simulink subsystem "SimulinkPlantModels"  (R2023b)
settings: Solver=VariableStepAuto  StartTime=0.0  StopTime=10.0  RelTol=1e-3
undefined symbols (not defined in the file): PlntTrnsfrCaseAxlSpdLock, PlntTrnsfrCaseTrqSplitRatio
libraries: simulink x2
settings Model: ModifiedByFormat=The MathWorks, Inc.  Creator=The MathWorks, Inc.  LastModifiedBy=The MathWorks, Inc.
settings DebuggingCC: SubsystemReferenceDiagnosticForUnitTest=warning

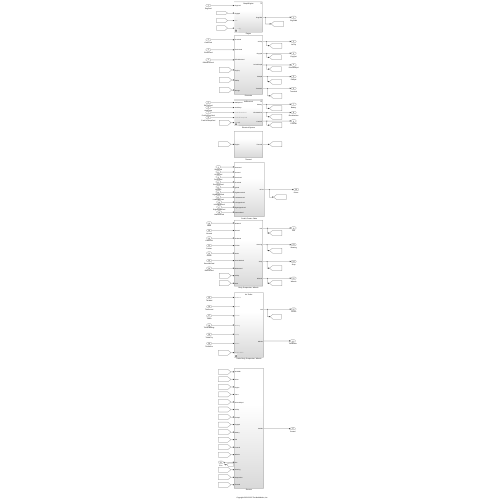
[thumbnail: Simulink's stored preview of the top-level diagram]
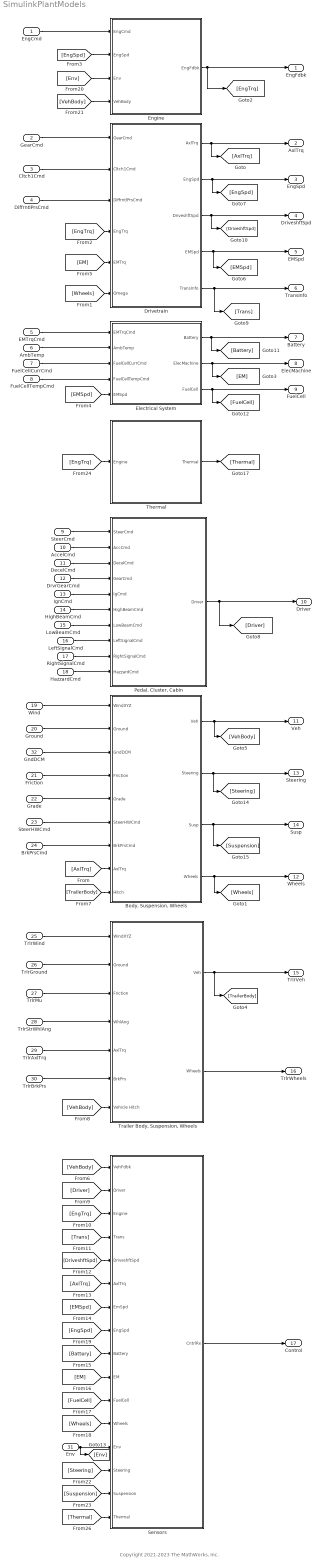
== system SimulinkPlantModels ==
  note: Copyright 2021-2023 The MathWorks, Inc.
  EngCmd : Inport
  GearCmd : Inport  Port=2
  Cltch1Cmd : Inport  Port=3
  DiffrntlPrsCmd : Inport  Port=4
  EMTrqCmd : Inport  Port=5
  AmbTemp : Inport  Port=6
  FuelCellCurrCmd : Inport  Port=7
  FuelCellTempCmd : Inport  Port=8
  SteerCmd : Inport  Port=9
  AccelCmd : Inport  Port=10
  DecelCmd : Inport  Port=11
  DrvrGearCmd : Inport  Port=12
  IgnCmd : Inport  Port=13
  HighBeamCmd : Inport  Port=14
  LowBeamCmd : Inport  Port=15
  LeftSignalCmd : Inport  Port=16
  RightSignalCmd : Inport  Port=17
  HazzardCmd : Inport  Port=18
  Wind : Inport  Port=19
  Ground : Inport  Port=20
  Friction : Inport  Port=21
  Grade : Inport  Port=22
  SteerHWCmd : Inport  Port=23
  BrkPrsCmd : Inport  Port=24
  TrlrWind : Inport  Port=25
  TrlrGround : Inport  Port=26
  TrlrMu : Inport  Port=27
  TrlrStrWhlAng : Inport  Port=28
  TrlrAxlTrq : Inport  Port=29
  TrlrBrkPrs : Inport  Port=30
  Env : Inport  Port=31
  GndDCM : Inport  Port=32
  "Body, Suspension, Wheels" : Subsystem  VariantControl=Lateral Vehicle Dynamics
  Drivetrain : Subsystem
  Electrical System : Subsystem  Variant=on  VariantChoicesSpecifier={'ElectricalSystem', 'NoElectrical'}  VariantControlMode=label  VariantControl=Choice  LabelModeActiveChoice=NoElectrical
  Engine : Subsystem  Variant=on  VariantChoicesSpecifier={'CiEngine', 'CiMappedEngine', 'FMUEngine', 'NoEngine', 'SiDLEngine', 'SiEngine', 'SiMappedEngine', 'SimpleEngine'}  VariantControlMode=label  LabelModeActiveChoice=SimpleEngine
  "Pedal, Cluster, Cabin" : Subsystem
  Sensors : Subsystem
  Thermal : Subsystem
  "Trailer Body, Suspension, Wheels" : Subsystem  Variant=on  VariantControlMode=label  LabelModeActiveChoice=No Trailer
  EngFdbk : Outport
  AxlTrq : Outport  Port=2
  EngSpd : Outport  Port=3
  DriveshftSpd : Outport  Port=4
  EMSpd : Outport  Port=5
  TransInfo : Outport  Port=6
  Battery : Outport  Port=7
  ElecMachine : Outport  Port=8
  FuelCell : Outport  Port=9
  Driver : Outport  Port=10
  Veh : Outport  Port=11
  Wheels : Outport  Port=12
  Steering : Outport  Port=13
  Susp : Outport  Port=14
  TrlrVeh : Outport  Port=15
  TrlrWheels : Outport  Port=16
  Control : Outport  Port=17
  wires:
  "Body, Suspension, Wheels"/2(Steering) -> [Steering], Steering/1
  [Suspension] -> Sensors/15(Suspension)
  "Body, Suspension, Wheels"/3(Susp) -> [Suspension], Susp/1
  [Steering] -> Sensors/14(Steering)
  Drivetrain/5(TransInfo) -> TransInfo/1, [Trans]
  Sensors/1(CntrlRx) -> Control/1
  Grade/1 -> "Body, Suspension, Wheels"/5(Grade)
  [EngTrq] -> Sensors/3(Engine)
  IgnCmd/1 -> "Pedal, Cluster, Cabin"/5(IgCmd)
  GndDCM/1 -> "Body, Suspension, Wheels"/3(GndDCM)
  Env/1 -> Sensors/13(Env), [Env]
  [EMSpd] -> Electrical System/5(EMSpd)
  EngCmd/1 -> Engine/1(EngCmd)
  Engine/1(EngFdbk) -> EngFdbk/1, [EngTrq]
  DiffrntlPrsCmd/1 -> Drivetrain/3(DiffrntlPrsCmd)
  [Env] -> Engine/3(Env)
  [VehBody] -> Engine/4(VehBody)
  [Battery] -> Sensors/9(Battery)
  [EngSpd] -> Sensors/8(EngSpd)
  [EngSpd] -> Engine/2(EngSpd)
  [Trans] -> Sensors/4(Trans)
  [Wheels] -> Sensors/12(Wheels)
  [EMSpd] -> Sensors/7(EmSpd)
  [EM] -> Sensors/10(EM)
  BrkPrsCmd/1 -> "Body, Suspension, Wheels"/7(BrkPrsCmd)
  FuelCellCurrCmd/1 -> Electrical System/3(FuelCellCurrCmd)
  [DriveshftSpd] -> Sensors/5(DriveshftSpd)
  [FuelCell] -> Sensors/11(FuelCell)
  [Driver] -> Sensors/2(Driver)
  "Trailer Body, Suspension, Wheels"/1(Veh) -> TrlrVeh/1, [TrailerBody]
  "Trailer Body, Suspension, Wheels"/2(Wheels) -> TrlrWheels/1
  Electrical System/2(ElecMachine) -> ElecMachine/1, [EM]
  [TrailerBody] -> "Body, Suspension, Wheels"/9(Hitch)
  "Body, Suspension, Wheels"/4(Wheels) -> [Wheels], Wheels/1
  "Pedal, Cluster, Cabin"/1(Driver) -> Driver/1, [Driver]
  Ground/1 -> "Body, Suspension, Wheels"/2(Ground)
  [VehBody] -> Sensors/1(VehFdbk)
  [Wheels] -> Drivetrain/6(Omega)
  GearCmd/1 -> Drivetrain/1(GearCmd)
  [EM] -> Drivetrain/5(EMTrq)
  Drivetrain/4(EMSpd) -> EMSpd/1, [EMSpd]
  [EngTrq] -> Drivetrain/4(EngTrq)
  AccelCmd/1 -> "Pedal, Cluster, Cabin"/2(AccCmd)
  EMTrqCmd/1 -> Electrical System/1(EMTrqCmd)
  Drivetrain/1(AxlTrq) -> AxlTrq/1, [AxlTrq]
  TrlrAxlTrq/1 -> "Trailer Body, Suspension, Wheels"/5(AxlTrq)
  Wind/1 -> "Body, Suspension, Wheels"/1(WindXYZ)
  TrlrStrWhlAng/1 -> "Trailer Body, Suspension, Wheels"/4(WhlAng)
  Friction/1 -> "Body, Suspension, Wheels"/4(Friction)
  FuelCellTempCmd/1 -> Electrical System/4(FuelCellTempCmd)
  [AxlTrq] -> "Body, Suspension, Wheels"/8(AxlTrq)
  TrlrWind/1 -> "Trailer Body, Suspension, Wheels"/1(WindXYZ)
  Drivetrain/3(DriveshftSpd) -> DriveshftSpd/1, [DriveshftSpd]
  SteerCmd/1 -> "Pedal, Cluster, Cabin"/1(SteerCmd)
  AmbTemp/1 -> Electrical System/2(AmbTemp)
  Cltch1Cmd/1 -> Drivetrain/2(Cltch1Cmd)
  DecelCmd/1 -> "Pedal, Cluster, Cabin"/3(DecelCmd)
  TrlrMu/1 -> "Trailer Body, Suspension, Wheels"/3(Friction)
  Drivetrain/2(EngSpd) -> EngSpd/1, [EngSpd]
  DrvrGearCmd/1 -> "Pedal, Cluster, Cabin"/4(GearCmd)
  [AxlTrq] -> Sensors/6(AxlTrq)
  SteerHWCmd/1 -> "Body, Suspension, Wheels"/6(SteerHWCmd)
  TrlrBrkPrs/1 -> "Trailer Body, Suspension, Wheels"/6(BrkPrs)
  [VehBody] -> "Trailer Body, Suspension, Wheels"/7(Vehicle Hitch)
  "Body, Suspension, Wheels"/1(Veh) -> Veh/1, [VehBody]
  Electrical System/3(FuelCell) -> FuelCell/1, [FuelCell]
  TrlrGround/1 -> "Trailer Body, Suspension, Wheels"/2(Ground)
  Electrical System/1(Battery) -> Battery/1, [Battery]
  Thermal/1(Thermal) -> [Thermal]
  [EngTrq] -> Thermal/1(Engine)
  [Thermal] -> Sensors/16(Thermal)
  RightSignalCmd/1 -> "Pedal, Cluster, Cabin"/9(RightSignalCmd)
  LowBeamCmd/1 -> "Pedal, Cluster, Cabin"/7(LowBeamCmd)
  HighBeamCmd/1 -> "Pedal, Cluster, Cabin"/6(HighBeamCmd)
  HazzardCmd/1 -> "Pedal, Cluster, Cabin"/10(HazzardCmd)
  LeftSignalCmd/1 -> "Pedal, Cluster, Cabin"/8(LeftSignalCmd)

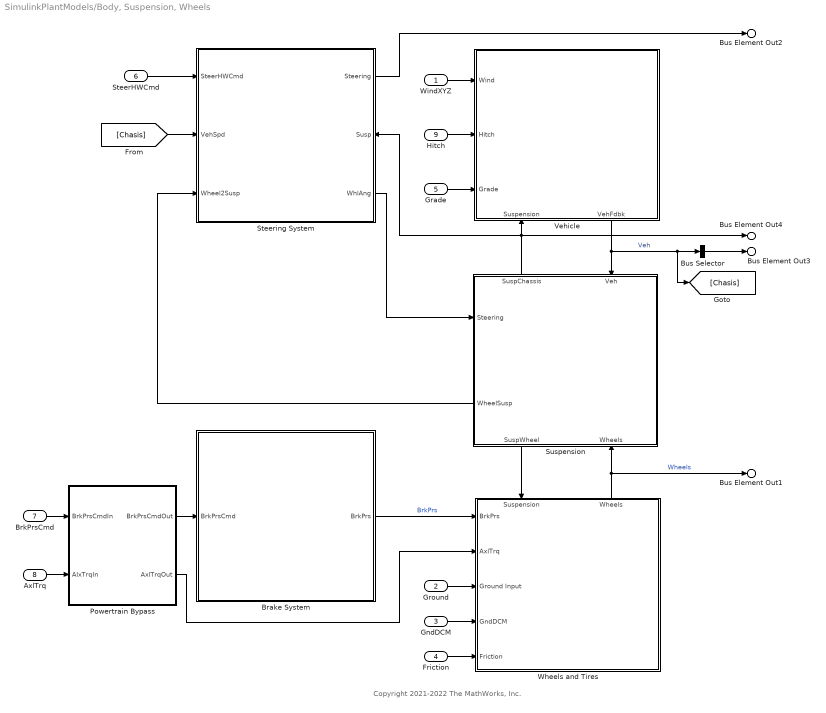
== system SimulinkPlantModels/Body, Suspension, Wheels ==
  note: Copyright 2021-2022 The MathWorks, Inc.
  WindXYZ : Inport  Unit=m/s  PortDimensions=3
  Ground : Inport  Port=2  Unit=m  PortDimensions=4
  GndDCM : Inport  Port=3
  Friction : Inport  Port=4  Unit=1  PortDimensions=4
  Grade : Inport  Port=5
  SteerHWCmd : Inport  Port=6  Unit=rad
  BrkPrsCmd : Inport  Port=7  PortDimensions=4
  AxlTrq : Inport  Port=8  Unit=N*m  PortDimensions=4
  Hitch : Inport  Port=9
  Brake System : Subsystem  Variant=on  VariantControlMode=label  VariantControl=Choice  LabelModeActiveChoice=BrakingHydraulics
      mask Display: disp('Brake System');
  Bus Selector : BusSelector  OutputSignals=InertFrm,BdyFrm  OutputAsBus=on
  Powertrain Bypass : Subsystem  Variant=on  VariantControlMode=label  VariantControl=Choice  LabelModeActiveChoice=Pass Through
  Steering System : Subsystem  Variant=on  VariantChoicesSpecifier={'DynamicSteering', 'KinematicSteering', 'MappedSteering', 'NoSteering', 'SteeringSystem'}  VariantControlMode=label  VariantControl=0  LabelModeActiveChoice=NoSteering
      settings: PortSchema="{\"entries\":[{\"content\":{\"sides\":[{\"content\":{\"connectorIds\":[\"In1\",\"In2\",\"In3\"]},\"type\":\"ConnectorPlacement.EquallySpacedRectSide\",\"uuid\":\"f4eae9a1-ee72-4894-9c3f-d81ee40fba89\"},{\"content\":{\"connectorIds\":[\"Out1\",\"In4\",\"Out2\"],\"side\":\"RIGHT\"},\"type\":\"ConnectorPlacement.EquallySpacedRectSide\",\"uuid\":\"c62a78d9-dc5d-4f96-a554-c82d7fa22a9e\"},{\"content\":{\"connectorIds\":[],\"side\":\"TOP\"},\"type\":\"ConnectorPlacement.EquallySpacedRectSide\",\"uuid\":\"38f3851a-1d1e-4a2b-8c09-8e5c8dcc7723\"}]},\"type\":\"ConnectorPlacement.EquallySpacedConnector\",\"uuid\":\"9f269846-92fa-4948-bc2b-71154f41fdde\"}],\"packageUris\":[\"http://schema.mathworks.com/mf0/Connector/R2020b\"],\"version\":\"1.0\"}"
      mask Display: disp('Steering System');
  Suspension : Subsystem  Variant=on  VariantChoicesSpecifier={'KinematicsComplianceIndependentSuspension', 'KinematicsComplianceTwistBeamSuspension', 'MacPhersonFrontSuspensionSolidAxleRearSuspension', 'NoSuspension'}  VariantControlMode=label  VariantControl=Choice  LabelModeActiveChoice=NoSuspension
      settings: PortSchema="{\"entries\":[{\"content\":{\"sides\":[{\"content\":{\"connectorIds\":[\"In1\",\"Out3\"]},\"type\":\"ConnectorPlacement.EquallySpacedRectSide\",\"uuid\":\"0a9265e3-f55e-4b74-9b74-681dc9522591\"},{\"content\":{\"connectorIds\":[],\"side\":\"RIGHT\"},\"type\":\"ConnectorPlacement.EquallySpacedRectSide\",\"uuid\":\"92df639a-7bc2-4e90-97ea-0cb216e2f16a\"},{\"content\":{\"connectorIds\":[\"Out2\",\"In2\"],\"side\":\"TOP\"},\"type\":\"ConnectorPlacement.EquallySpacedRectSide\",\"uuid\":\"2064b6cb-c7a8-4cfb-82de-a07750d990cb\"},{\"content\":{\"connectorIds\":[\"Out1\",\"In3\"],\"side\":\"BOTTOM\"},\"type\":\"ConnectorPlacement.EquallySpacedRectSide\",\"uuid\":\"169bd4e6-c3fe-4e36-acea-c25875014463\"}]},\"type\":\"ConnectorPlacement.EquallySpacedConnector\",\"uuid\":\"e0b50182-0637-4594-80e7-4ddd0df85797\"}],\"packageUris\":[\"http://schema.mathworks.com/mf0/Connector/R2020b\"],\"version\":\"1.0\"}"
      mask Display: disp('Suspension');
  Vehicle : Subsystem  Variant=on  VariantChoicesSpecifier={'VehicleBody1DOFLongitudinal', 'VehicleBody3DOFLongitudinal', 'VehicleBody6DOF'}  VariantControlMode=label  VariantControl=Choice  LabelModeActiveChoice=VehicleBody3DOFLongitudinal
      settings: PortSchema="{\"entries\":[{\"content\":{\"sides\":[{\"content\":{\"connectorIds\":[\"In1\",\"In2\",\"In3\"]},\"type\":\"ConnectorPlacement.EquallySpacedRectSide\",\"uuid\":\"0a9265e3-f55e-4b74-9b74-681dc9522591\"},{\"content\":{\"connectorIds\":[],\"side\":\"RIGHT\"},\"type\":\"ConnectorPlacement.EquallySpacedRectSide\",\"uuid\":\"92df639a-7bc2-4e90-97ea-0cb216e2f16a\"},{\"content\":{\"connectorIds\":[],\"side\":\"TOP\"},\"type\":\"ConnectorPlacement.EquallySpacedRectSide\",\"uuid\":\"2064b6cb-c7a8-4cfb-82de-a07750d990cb\"},{\"content\":{\"connectorIds\":[\"In4\",\"Out1\"],\"side\":\"BOTTOM\"},\"type\":\"ConnectorPlacement.EquallySpacedRectSide\",\"uuid\":\"2b34afca-0a88-43db-924f-6476183b84bd\"}]},\"type\":\"ConnectorPlacement.EquallySpacedConnector\",\"uuid\":\"e0b50182-0637-4594-80e7-4ddd0df85797\"}],\"packageUris\":[\"http://schema.mathworks.com/mf0/Connector/R2020b\"],\"version\":\"1.0\"}"
      mask Display: disp('Vehicle Body');
  Wheels and Tires : Subsystem  Variant=on  VariantChoicesSpecifier={'CombinedSlipTiresLongitudinal', 'DugoffTires', 'FialaTires', 'MFTires', 'MFTiresLongitudinal'}  VariantControlMode=label  VariantControl=Choice  LabelModeActiveChoice=MFTiresLongitudinal
      settings: PortSchema="{\"entries\":[{\"content\":{\"sides\":[{\"content\":{\"connectorIds\":[\"In1\",\"In2\",\"In3\",\"In4\",\"In5\"]},\"type\":\"ConnectorPlacement.EquallySpacedRectSide\",\"uuid\":\"fdb4d4cd-d0c0-42d9-b073-775af31e96a1\"},{\"content\":{\"connectorIds\":[],\"side\":\"RIGHT\"},\"type\":\"ConnectorPlacement.EquallySpacedRectSide\",\"uuid\":\"04106ddf-9917-4cd4-b177-ae763d642686\"},{\"content\":{\"connectorIds\":[\"In6\",\"Out1\"],\"side\":\"TOP\"},\"type\":\"ConnectorPlacement.EquallySpacedRectSide\",\"uuid\":\"568bf95c-0e25-4c45-a134-c198357b75be\"}]},\"type\":\"ConnectorPlacement.EquallySpacedConnector\",\"uuid\":\"4f44df5e-0d14-43ea-934e-2abe86546e95\"}],\"packageUris\":[\"http://schema.mathworks.com/mf0/Connector/R2020b\"],\"version\":\"1.0\"}"
      mask Display: disp('Wheels and Tires');
  Bus Element Out3 : Outport  PortName=Veh
  Bus Element Out2 : Outport  Port=2  PortName=Steering
  Bus Element Out4 : Outport  Port=3  PortName=Susp
  Bus Element Out1 : Outport  Port=4  PortName=Wheels
  wires:
  GndDCM/1 -> Wheels and Tires/4(GndDCM)
  Friction/1 -> Wheels and Tires/5(Friction)
  Powertrain Bypass/2(AxlTrqOut) -> Wheels and Tires/2(AxlTrq)
  Ground/1 -> Wheels and Tires/3(Ground Input)
  Grade/1 -> Vehicle/3(Grade)
  Wheels and Tires/1(Wheels) -> Bus Element Out1/1, Suspension/3(Wheels)  "Wheels"
  Suspension/1(SuspWheel) -> Wheels and Tires/6(Suspension)
  Brake System/1(BrkPrs) -> Wheels and Tires/1(BrkPrs)  "BrkPrs"
  Vehicle/1(VehFdbk) -> [Chasis], Bus Selector/1, Suspension/2(Veh)  "Veh"
  Hitch/1 -> Vehicle/2(Hitch)
  WindXYZ/1 -> Vehicle/1(Wind)
  Suspension/2(SuspChassis) -> Steering System/4(Susp), Bus Element Out4/1, Vehicle/4(Suspension)
  Steering System/2(WhlAng) -> Suspension/1(Steering)
  BrkPrsCmd/1 -> Powertrain Bypass/1(BrkPrsCmdIn)
  Bus Selector/1 -> Bus Element Out3/1
  [Chasis] -> Steering System/2(VehSpd)
  SteerHWCmd/1 -> Steering System/1(SteerHWCmd)
  Steering System/1(Steering) -> Bus Element Out2/1
  Powertrain Bypass/1(BrkPrsCmdOut) -> Brake System/1(BrkPrsCmd)
  AxlTrq/1 -> Powertrain Bypass/2(AlxTrqIn)
  Suspension/3(WheelSusp) -> Steering System/3(Wheel2Susp)

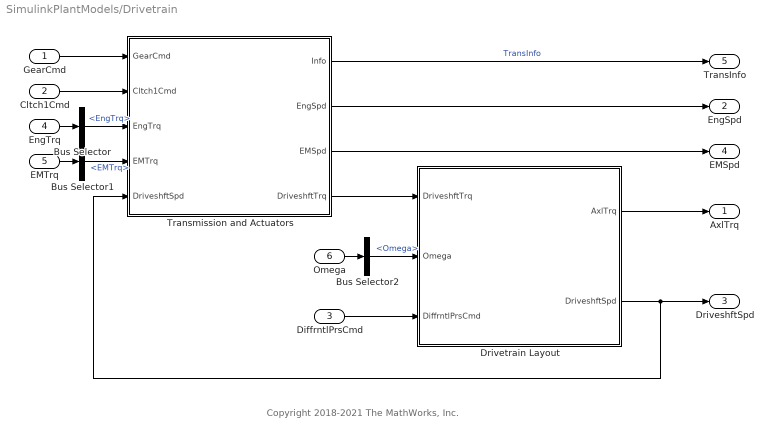
== system SimulinkPlantModels/Drivetrain ==
  note: Copyright 2018-2021 The MathWorks, Inc.
  GearCmd : Inport
  Cltch1Cmd : Inport  Port=2
  DiffrntlPrsCmd : Inport  Port=3
  EngTrq : Inport  Port=4
  EMTrq : Inport  Port=5
  Omega : Inport  Port=6
  Bus Selector : BusSelector  OutputSignals=EngTrq
  Bus Selector1 : BusSelector  OutputSignals=EMTrq
  Bus Selector2 : BusSelector  OutputSignals=Wheels.Omega
  Drivetrain Layout : Subsystem  VariantControl=New
  Transmission and Actuators : Subsystem  Variant=on  VariantChoicesSpecifier={'BEV1EM', 'BEV2EM', 'BEV3EM', 'BEV4EM', 'ConventionalVehicle', 'HEVIPS', 'HEVMM', 'HEVP0', 'HEVP1', 'HEVP2', 'HEVP3', 'HEVP4'}  VariantControlMode=label  LabelModeActiveChoice=ConventionalVehicle
  AxlTrq : Outport  VectorParamsAs1DForOutWhenUnconnected=off
  EngSpd : Outport  Port=2  Unit=rad/s  VectorParamsAs1DForOutWhenUnconnected=off
  DriveshftSpd : Outport  Port=3  VectorParamsAs1DForOutWhenUnconnected=off
  EMSpd : Outport  Port=4  Unit=rad/s  VectorParamsAs1DForOutWhenUnconnected=off
  TransInfo : Outport  Port=5  VectorParamsAs1DForOutWhenUnconnected=off
  wires:
  Transmission and Actuators/1(Info) -> TransInfo/1  "TransInfo"
  DiffrntlPrsCmd/1 -> Drivetrain Layout/3(DiffrntlPrsCmd)
  Cltch1Cmd/1 -> Transmission and Actuators/2(Cltch1Cmd)
  Drivetrain Layout/2(DriveshftSpd) -> DriveshftSpd/1, Transmission and Actuators/5(DriveshftSpd)
  GearCmd/1 -> Transmission and Actuators/1(GearCmd)
  Drivetrain Layout/1(AxlTrq) -> AxlTrq/1
  Transmission and Actuators/2(EngSpd) -> EngSpd/1
  Transmission and Actuators/3(EMSpd) -> EMSpd/1
  Transmission and Actuators/4(DriveshftTrq) -> Drivetrain Layout/1(DriveshftTrq)
  EngTrq/1 -> Bus Selector/1
  Bus Selector/1 -> Transmission and Actuators/3(EngTrq)  "<EngTrq>"
  EMTrq/1 -> Bus Selector1/1
  Bus Selector1/1 -> Transmission and Actuators/4(EMTrq)  "<EMTrq>"
  Omega/1 -> Bus Selector2/1
  Bus Selector2/1 -> Drivetrain Layout/2(Omega)  "<Omega>"

== system SimulinkPlantModels/Electrical System ==
  EMTrqCmd : Inport
  AmbTemp : Inport  Port=2
  FuelCellCurrCmd : Inport  Port=3
  FuelCellTempCmd : Inport  Port=4
  EMSpd : Inport  Port=5
  ElectricalSystem : Subsystem  VariantControl=ElectricalSystem  ReferencedSubsystem=ElectricalSystem
  NoElectrical : Subsystem  VariantControl=NoElectrical  ReferencedSubsystem=NoElectrical
  Battery : Outport
  ElecMachine : Outport  Port=2
  FuelCell : Outport  Port=3

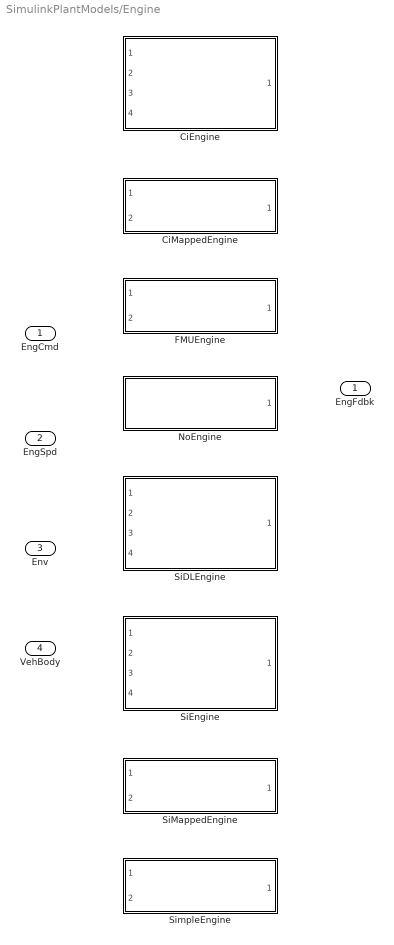
== system SimulinkPlantModels/Engine ==
  EngCmd : Inport
  EngSpd : Inport  Port=2
  Env : Inport  Port=3
  VehBody : Inport  Port=4
  CiEngine : Subsystem  VariantControl=CiEngine  ReferencedSubsystem=CiEngine
  CiMappedEngine : Subsystem  VariantControl=CiMappedEngine  ReferencedSubsystem=CiMappedEngine
  FMUEngine : Subsystem  VariantControl=FMUEngine  ReferencedSubsystem=FMUEngine
  NoEngine : Subsystem  VariantControl=NoEngine  ReferencedSubsystem=NoEngine
  SiDLEngine : Subsystem  VariantControl=SiDLEngine  ReferencedSubsystem=SiDLEngine
  SiEngine : Subsystem  VariantControl=SiEngine  ReferencedSubsystem=SiEngine
  SiMappedEngine : Subsystem  VariantControl=SiMappedEngine  ReferencedSubsystem=SiMappedEngine
  SimpleEngine : Subsystem  VariantControl=SimpleEngine  ReferencedSubsystem=SimpleEngine
  EngFdbk : Outport  VectorParamsAs1DForOutWhenUnconnected=off

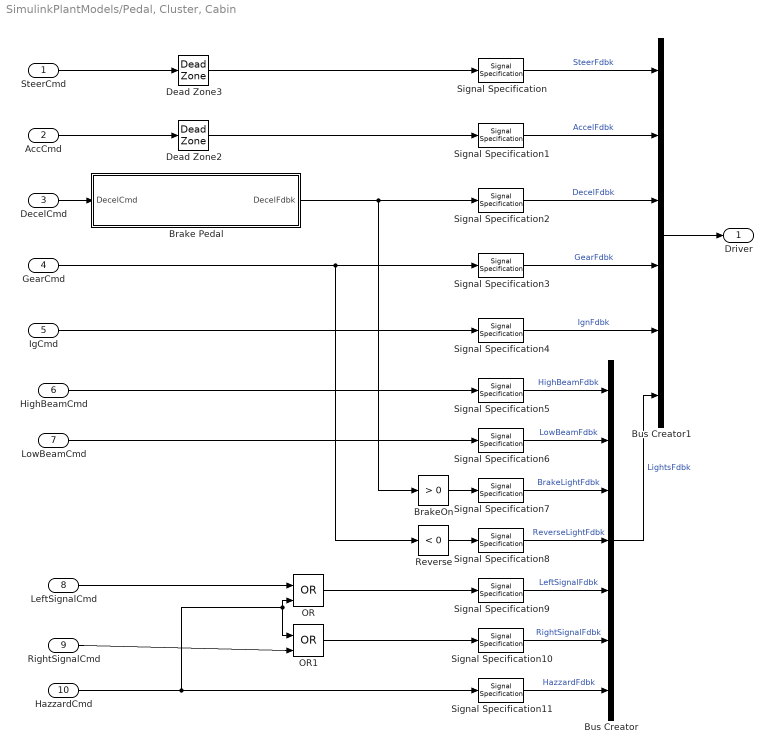
== system SimulinkPlantModels/Pedal, Cluster, Cabin ==
  SteerCmd : Inport
  AccCmd : Inport  Port=2
  DecelCmd : Inport  Port=3
  GearCmd : Inport  Port=4
  IgCmd : Inport  Port=5
  HighBeamCmd : Inport  Port=6
  LowBeamCmd : Inport  Port=7
  LeftSignalCmd : Inport  Port=8
  RightSignalCmd : Inport  Port=9
  HazzardCmd : Inport  Port=10
  Brake Pedal : Subsystem
  BrakeOn : simulink/Logic and Bit Operations/Compare To Constant  relop=>  const=0  OutDataTypeStr=boolean  ZeroCross=off
  Bus Creator : BusCreator  Inputs=7
  Bus Creator1 : BusCreator  Inputs=6
  Dead Zone2 : DeadZone  LowerValue=0  UpperValue=.01  ZeroCross=off
  Dead Zone3 : DeadZone  LowerValue=-.01  UpperValue=.01  ZeroCross=off
  OR : Logic  Operator=OR  IconShape=distinctive  AllPortsSameDT=off  OutDataTypeStr=boolean
  OR1 : Logic  Operator=OR  IconShape=distinctive  AllPortsSameDT=off  OutDataTypeStr=boolean
  Reverse : simulink/Logic and Bit Operations/Compare To Constant  relop=<  const=0  OutDataTypeStr=boolean  ZeroCross=off
  Signal Specification : SignalSpecification  Unit=rad
  Signal Specification{1..11} (11 alike) : SignalSpecification  Unit=1
  Driver : Outport
  wires:
  Signal Specification9/1 -> Bus Creator/5  "LeftSignalFdbk"
  Signal Specification11/1 -> Bus Creator/7  "HazzardFdbk"
  Signal Specification10/1 -> Bus Creator/6  "RightSignalFdbk"
  Signal Specification8/1 -> Bus Creator/4  "ReverseLightFdbk"
  Signal Specification7/1 -> Bus Creator/3  "BrakeLightFdbk"
  Signal Specification6/1 -> Bus Creator/2  "LowBeamFdbk"
  Signal Specification5/1 -> Bus Creator/1  "HighBeamFdbk"
  Bus Creator/1 -> Bus Creator1/6  "LightsFdbk"
  RightSignalCmd/1 -> OR1/2
  LowBeamCmd/1 -> Signal Specification6/1
  HazzardCmd/1 -> OR1/1, OR/2, Signal Specification11/1
  LeftSignalCmd/1 -> OR/1
  Reverse/1 -> Signal Specification8/1
  OR/1 -> Signal Specification9/1
  OR1/1 -> Signal Specification10/1
  BrakeOn/1 -> Signal Specification7/1
  HighBeamCmd/1 -> Signal Specification5/1
  Dead Zone3/1 -> Signal Specification/1
  Signal Specification1/1 -> Bus Creator1/2  "AccelFdbk"
  Signal Specification4/1 -> Bus Creator1/5  "IgnFdbk"
  Brake Pedal/1(DecelFdbk) -> Signal Specification2/1, BrakeOn/1
  Signal Specification/1 -> Bus Creator1/1  "SteerFdbk"
  Signal Specification2/1 -> Bus Creator1/3  "DecelFdbk"
  GearCmd/1 -> Signal Specification3/1, Reverse/1
  Bus Creator1/1 -> Driver/1
  IgCmd/1 -> Signal Specification4/1
  Signal Specification3/1 -> Bus Creator1/4  "GearFdbk"
  Dead Zone2/1 -> Signal Specification1/1
  SteerCmd/1 -> Dead Zone3/1
  AccCmd/1 -> Dead Zone2/1
  DecelCmd/1 -> Brake Pedal/1(DecelCmd)

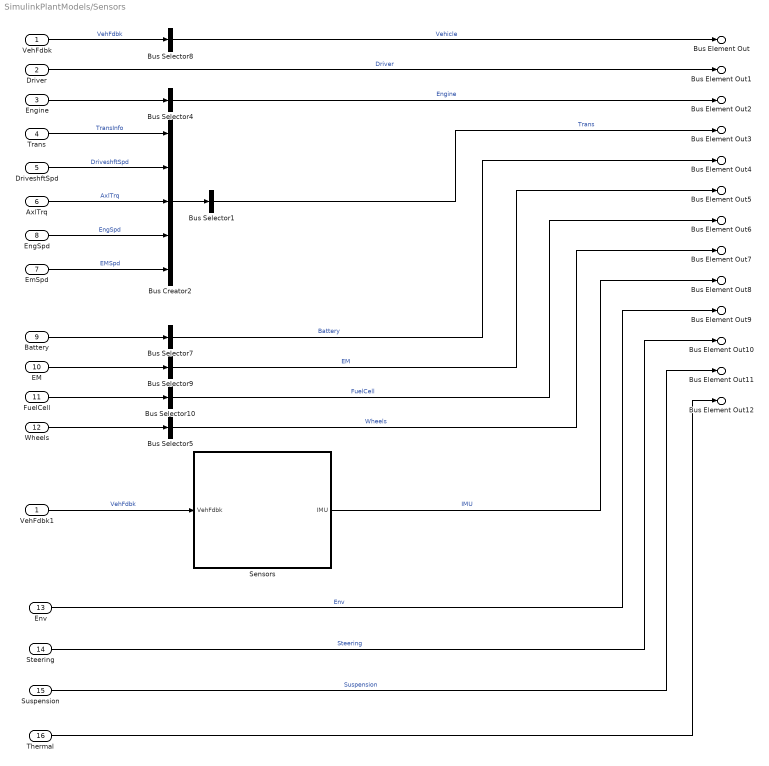
== system SimulinkPlantModels/Sensors ==
  VehFdbk : Inport
  Driver : Inport  Port=2
  Engine : Inport  Port=3
  Trans : Inport  Port=4
  DriveshftSpd : Inport  Port=5
  AxlTrq : Inport  Port=6
  EmSpd : Inport  Port=7
  EngSpd : Inport  Port=8
  Battery : Inport  Port=9
  EM : Inport  Port=10
  FuelCell : Inport  Port=11
  Wheels : Inport  Port=12
  Env : Inport  Port=13
  Steering : Inport  Port=14
  Suspension : Inport  Port=15
  Thermal : Inport  Port=16
  Bus Creator2 : BusCreator  Inputs=5
  Bus Selector1 : BusSelector  OutputSignals=TransInfo.Cltch1State,TransInfo.Cltch2State,DriveshftSpd,AxlTrq,EngSpd,EMSpd,TransInfo.TransInfo.Trans.TransGear  OutputAsBus=on
  Bus Selector10 : BusSelector  OutputSignals=FuelCellVolt,FuelCellCurr,H2Flw  OutputAsBus=on
  Bus Selector4 : BusSelector  OutputSignals=EngTrq,Map,Mat,ThrPosPct,WgAreaPct,IntkCamPhase,ExhCamPhase,TurboRackPos,EgrVlvAreaPct,VarCompRatioPos,IntkVlvLift,VarIntkRunLen,Afr,IntkSwirlVlvPos,TurboSpd,Iat,Ect,EgrVlvDeltaPrs,EgrVlvInTemp  OutputAsBus=on
  Bus Selector5 : BusSelector  OutputSignals=Wheels.BrkPrs,Wheels.Kappa,Wheels.Alpha,Wheels.Omega  OutputAsBus=on
  Bus Selector7 : BusSelector  OutputSignals=BattSoc,BattVolt,BattCurr,BattPwr,BMSSensors  OutputAsBus=on
  Bus Selector8 : BusSelector  OutputSignals=BdyFrm.Cg.Vel.xdot,BdyFrm.Cg.Acc.ax,BdyFrm.Cg.Acc.xddot  OutputAsBus=on
  Bus Selector9 : BusSelector  OutputSignals=EMTrq,EMPwrElec  OutputAsBus=on
  Sensors : Subsystem  Variant=on  VariantChoicesSpecifier={'IMUSensor', 'NoIMUSensor'}  VariantControlMode=label  VariantControl=Choice  LabelModeActiveChoice=NoIMUSensor
  VehFdbk1 : InportShadow
  Bus Element Out : Outport  PortName=CntrlRx  Element=Vehicle
  Bus Element Out1 : Outport  PortName=CntrlRx  Element=Driver
  Bus Element Out2 : Outport  PortName=CntrlRx  Element=Engine
  Bus Element Out3 : Outport  PortName=CntrlRx  Element=Trans
  Bus Element Out4 : Outport  PortName=CntrlRx  Element=Battery
  Bus Element Out5 : Outport  PortName=CntrlRx  Element=EM
  Bus Element Out6 : Outport  PortName=CntrlRx  Element=FuelCell
  Bus Element Out7 : Outport  PortName=CntrlRx  Element=Wheels
  Bus Element Out8 : Outport  PortName=CntrlRx  Element=IMU
  Bus Element Out9 : Outport  PortName=CntrlRx  Element=Env
  Bus Element Out10 : Outport  PortName=CntrlRx  Element=Steering
  Bus Element Out11 : Outport  PortName=CntrlRx  Element=Suspension
  Bus Element Out12 : Outport  PortName=CntrlRx  Element=Thermal
  wires:
  Thermal/1 -> Bus Element Out12/1
  Suspension/1 -> Bus Element Out11/1  "Suspension"
  Steering/1 -> Bus Element Out10/1  "Steering"
  Bus Selector5/1 -> Bus Element Out7/1  "Wheels"
  Bus Selector7/1 -> Bus Element Out4/1  "Battery"
  Bus Selector8/1 -> Bus Element Out/1  "Vehicle"
  Bus Selector9/1 -> Bus Element Out5/1  "EM"
  Bus Selector10/1 -> Bus Element Out6/1  "FuelCell"
  Bus Selector4/1 -> Bus Element Out2/1  "Engine"
  VehFdbk/1 -> Bus Selector8/1  "VehFdbk"
  Engine/1 -> Bus Selector4/1
  DriveshftSpd/1 -> Bus Creator2/2  "DriveshftSpd"
  AxlTrq/1 -> Bus Creator2/3  "AxlTrq"
  EmSpd/1 -> Bus Creator2/5  "EMSpd"
  Battery/1 -> Bus Selector7/1
  EM/1 -> Bus Selector9/1
  FuelCell/1 -> Bus Selector10/1
  Wheels/1 -> Bus Selector5/1
  VehFdbk1/1 -> Sensors/1(VehFdbk)  "VehFdbk"
  Sensors/1(IMU) -> Bus Element Out8/1  "IMU"
  Driver/1 -> Bus Element Out1/1  "Driver"
  Env/1 -> Bus Element Out9/1  "Env"
  EngSpd/1 -> Bus Creator2/4  "EngSpd"
  Trans/1 -> Bus Creator2/1  "TransInfo"
  Bus Creator2/1 -> Bus Selector1/1
  Bus Selector1/1 -> Bus Element Out3/1  "Trans"

== system SimulinkPlantModels/Thermal ==
  Engine : Inport
  Electrical Cooling : Subsystem  Variant=on  VariantControlMode=label  LabelModeActiveChoice=No Thermal Effect
  Terminator : Terminator
  Thermal : Outport
  wires:
  Electrical Cooling/1(Thermal) -> Thermal/1
  Engine/1 -> Terminator/1

== system SimulinkPlantModels/Trailer Body, Suspension, Wheels ==
  WindXYZ : Inport
  Ground : Inport  Port=2
  Friction : Inport  Port=3
  WhlAng : Inport  Port=4
  AxlTrq : Inport  Port=5
  BrkPrs : Inport  Port=6
  Vehicle Hitch : Inport  Port=7
  No Trailer : Subsystem  VariantControl=No Trailer
  One-Axle Trailer : Subsystem  VariantControl=One-Axle Trailer  ReferencedSubsystem=OneAxleTrailer
  Veh : Outport  VectorParamsAs1DForOutWhenUnconnected=off
  Wheels : Outport  Port=2  VectorParamsAs1DForOutWhenUnconnected=off

== system SimulinkPlantModels/Body, Suspension, Wheels/Brake System ==
  BrkPrsCmd : Inport
  BrakingHydraulics : Subsystem  VariantControl=BrakingHydraulics  ReferencedSubsystem=BrakingHydraulics
  BrkPrs : Outport

== system SimulinkPlantModels/Body, Suspension, Wheels/Powertrain Bypass ==
  BrkPrsCmdIn : Inport
  AlxTrqIn : Inport  Port=2
  External Signal Source : Subsystem  VariantControl=External Signal Source
  Pass Through : Subsystem  VariantControl=Pass Through
  BrkPrsCmdOut : Outport
  AxlTrqOut : Outport  Port=2

== system SimulinkPlantModels/Body, Suspension, Wheels/Steering System ==
  SteerHWCmd : Inport
  VehSpd : Inport  Port=2
  Wheel2Susp : Inport  Port=3
  Susp : Inport  Port=4
  DynamicSteering : Subsystem  VariantControl=DynamicSteering  ReferencedSubsystem=DynamicSteering
  KinematicSteering : Subsystem  VariantControl=KinematicSteering  ReferencedSubsystem=KinematicSteering
  MappedSteering : Subsystem  VariantControl=MappedSteering  ReferencedSubsystem=MappedSteering
  NoSteering : Subsystem  VariantControl=NoSteering  ReferencedSubsystem=NoSteering
  SteeringSystem : Subsystem  VariantControl=SteeringSystem  ReferencedSubsystem=SteeringSystem
  Steering : Outport
  WhlAng : Outport  Port=2  VectorParamsAs1DForOutWhenUnconnected=off

== system SimulinkPlantModels/Body, Suspension, Wheels/Suspension ==
  Steering : Inport
  Veh : Inport  Port=2
  Wheels : Inport  Port=3
  KinematicsComplianceIndependentSuspension : Subsystem  VariantControl=KinematicsComplianceIndependentSuspension  ReferencedSubsystem=KinematicsComplianceIndependentSuspension
  KinematicsComplianceTwistBeamSuspension : Subsystem  VariantControl=KinematicsComplianceTwistBeamSuspension  ReferencedSubsystem=KinematicsComplianceTwistBeamSuspension
  MacPhersonFrontSuspensionSolidAxleRearSuspension : Subsystem  VariantControl=MacPhersonFrontSuspensionSolidAxleRearSuspension  ReferencedSubsystem=MacPhersonFrontSuspensionSolidAxleRearSuspension
  NoSuspension : Subsystem  VariantControl=NoSuspension  ReferencedSubsystem=NoSuspension
  SuspWheel : Outport
  SuspChassis : Outport  Port=2
  WheelSusp : Outport  Port=3

== system SimulinkPlantModels/Body, Suspension, Wheels/Vehicle ==
  Wind : Inport
  Hitch : Inport  Port=2
  Grade : Inport  Port=3
  Suspension : Inport  Port=4
  VehicleBody1DOFLongitudinal : Subsystem  VariantControl=VehicleBody1DOFLongitudinal  ReferencedSubsystem=VehicleBody1DOFLongitudinal
  VehicleBody3DOFLongitudinal : Subsystem  VariantControl=VehicleBody3DOFLongitudinal  ReferencedSubsystem=VehicleBody3DOFLongitudinal
  VehicleBody6DOF : Subsystem  VariantControl=VehicleBody6DOF  ReferencedSubsystem=VehicleBody6DOF
  VehFdbk : Outport

== system SimulinkPlantModels/Body, Suspension, Wheels/Wheels and Tires ==
  BrkPrs : Inport
  AxlTrq : Inport  Port=2
  Ground Input : Inport  Port=3
  GndDCM : Inport  Port=4
  Friction : Inport  Port=5
  Suspension : Inport  Port=6
  CombinedSlipTiresLongitudinal : Subsystem  VariantControl=CombinedSlipTiresLongitudinal  ReferencedSubsystem=CombinedSlipTiresLongitudinal
  DugoffTires : Subsystem  VariantControl=DugoffTires  ReferencedSubsystem=DugoffTires
  FialaTires : Subsystem  VariantControl=FialaTires  ReferencedSubsystem=FialaTires
  MFTires : Subsystem  VariantControl=MFTires  ReferencedSubsystem=MFTires
  MFTiresLongitudinal : Subsystem  VariantControl=MFTiresLongitudinal  ReferencedSubsystem=MFTiresLongitudinal
  Wheels : Outport

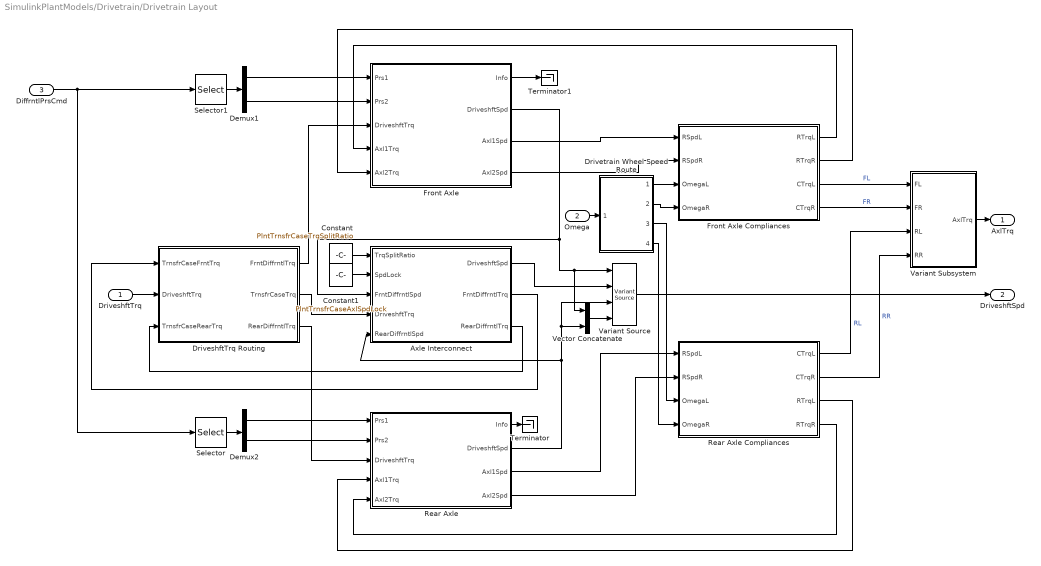
== system SimulinkPlantModels/Drivetrain/Drivetrain Layout ==
  DriveshftTrq : Inport
  Omega : Inport  Port=2
  DiffrntlPrsCmd : Inport  Port=3
  Axle Interconnect : Subsystem  Variant=on  VariantChoicesSpecifier={'NoInterconnect', 'TransferCase'}  VariantControlMode=label  VariantControl=Choice  LabelModeActiveChoice=NoInterconnect
  Constant : Constant  Value=PlntTrnsfrCaseTrqSplitRatio  SampleTime=-1
  Constant1 : Constant  Value=PlntTrnsfrCaseAxlSpdLock  SampleTime=-1
  Demux1 : Demux  Outputs=2
  Demux2 : Demux  Outputs=2
  DriveshftTrq Routing : Subsystem  Variant=on  VariantChoicesSpecifier={'FourActuatorAWD', 'OneActuatorAWD', 'OneActuatorFWD', 'OneActuatorRWD', 'ThreeActuatorAWD2EMFront', 'ThreeActuatorAWD2EMRear', 'TwoActuatorAWD'}  VariantControlMode=label  VariantControl=Choice  LabelModeActiveChoice=OneActuatorFWD
  Drivetrain Wheel Speed Route : Subsystem  Variant=on  VariantControlMode=label  LabelModeActiveChoice=Bus
  Front Axle : Subsystem  Variant=on  VariantChoicesSpecifier={'ActiveDifferential', 'DualEMDriveFront', 'LimitedSlipDifferential', 'NoDifferential', 'OpenDifferential'}  VariantControlMode=label  VariantControl=Choice  LabelModeActiveChoice=OpenDifferential
  Front Axle Compliances : Subsystem  Variant=on  VariantChoicesSpecifier={'AxleCompliances', 'NoAxleCompliances'}  VariantControlMode=label  VariantControl=Choice  LabelModeActiveChoice=AxleCompliances
  Rear Axle : Subsystem  Variant=on  VariantChoicesSpecifier={'ActiveDifferential', 'DualEMDriveRear', 'LimitedSlipDifferential', 'NoDifferential', 'OpenDifferential'}  VariantControlMode=label  VariantControl=Choice  LabelModeActiveChoice=NoDifferential
  Rear Axle Compliances : Subsystem  Variant=on  VariantChoicesSpecifier={'AxleCompliances', 'NoAxleCompliances'}  VariantControlMode=label  VariantControl=Choice  LabelModeActiveChoice=NoAxleCompliances
  Selector : Selector  InputPortWidth=4  IndexOptions=Index vector (dialog)  Indices=[3 4]  OutputSizes=1
  Selector1 : Selector  InputPortWidth=4  IndexOptions=Index vector (dialog)  Indices=[1 2]  OutputSizes=1
  Terminator : Terminator
  Terminator1 : Terminator
  Variant Source : VariantSource  VariantControlMode=label  LabelModeActiveChoice=One Actuator FWD
  Variant Subsystem : Subsystem  Variant=on  VariantControlMode=label  LabelModeActiveChoice=TwoAxleOutput
  Vector Concatenate : Concatenate
  AxlTrq : Outport  VectorParamsAs1DForOutWhenUnconnected=off
  DriveshftSpd : Outport  Port=2  VectorParamsAs1DForOutWhenUnconnected=off
  wires:
  Selector/1 -> Demux2/1
  Demux2/1 -> Rear Axle/1(Prs1)
  Demux2/2 -> Rear Axle/2(Prs2)
  Demux1/2 -> Front Axle/2(Prs2)
  Demux1/1 -> Front Axle/1(Prs1)
  Selector1/1 -> Demux1/1
  Omega/1 -> Drivetrain Wheel Speed Route/1(Omega)
  Front Axle Compliances/1(RTrqL) -> Front Axle/4(Axl1Trq)
  Front Axle Compliances/2(RTrqR) -> Front Axle/5(Axl2Trq)
  Front Axle/4(Axl2Spd) -> Front Axle Compliances/2(RSpdR)
  Front Axle/3(Axl1Spd) -> Front Axle Compliances/1(RSpdL)
  DiffrntlPrsCmd/1 -> Selector/1, Selector1/1
  Rear Axle/2(DriveshftSpd) -> Vector Concatenate/2, Variant Source/3, Axle Interconnect/5(RearDiffrntlSpd)
  Front Axle/2(DriveshftSpd) -> Axle Interconnect/3(FrntDiffrntlSpd), Variant Source/1, Vector Concatenate/1
  DriveshftTrq/1 -> DriveshftTrq Routing/2(DriveshftTrq)
  DriveshftTrq Routing/1(FrntDiffrntlTrq) -> Front Axle/3(DriveshftTrq)
  DriveshftTrq Routing/3(RearDiffrntlTrq) -> Rear Axle/3(DriveshftTrq)
  Rear Axle/1(Info) -> Terminator/1
  Front Axle/1(Info) -> Terminator1/1
  Variant Source/1 -> DriveshftSpd/1
  DriveshftTrq Routing/2(TrnsfrCaseTrq) -> Axle Interconnect/4(DriveshftTrq)
  Axle Interconnect/1(DriveshftSpd) -> Variant Source/2
  Axle Interconnect/2(FrntDiffrntlTrq) -> DriveshftTrq Routing/1(TrnsfrCaseFrntTrq)
  Axle Interconnect/3(RearDiffrntlTrq) -> DriveshftTrq Routing/3("TrnsfrCaseRearTrq ")
  Vector Concatenate/1 -> Variant Source/4
  Rear Axle/3(Axl1Spd) -> Rear Axle Compliances/1(RSpdL)
  Rear Axle/4(Axl2Spd) -> Rear Axle Compliances/2(RSpdR)
  Rear Axle Compliances/3(RTrqL) -> Rear Axle/4(Axl1Trq)
  Rear Axle Compliances/4(RTrqR) -> Rear Axle/5(Axl2Trq)
  Constant/1 -> Axle Interconnect/1(TrqSplitRatio)
  Constant1/1 -> Axle Interconnect/2(SpdLock)
  Drivetrain Wheel Speed Route/1(Omega_LF) -> Front Axle Compliances/3(OmegaL)
  Drivetrain Wheel Speed Route/2(Omega_RF) -> Front Axle Compliances/4(OmegaR)
  Drivetrain Wheel Speed Route/3(Omega_LR) -> Rear Axle Compliances/3(OmegaL)
  Drivetrain Wheel Speed Route/4(Omega_RR) -> Rear Axle Compliances/4(OmegaR)
  Front Axle Compliances/3(CTrqL) -> Variant Subsystem/1(FL)  "FL"
  Front Axle Compliances/4(CTrqR) -> Variant Subsystem/2(FR)  "FR"
  Rear Axle Compliances/1(CTrqL) -> Variant Subsystem/3(RL)  "RL"
  Rear Axle Compliances/2(CTrqR) -> Variant Subsystem/4(RR)  "RR"
  Variant Subsystem/1(AxlTrq) -> AxlTrq/1

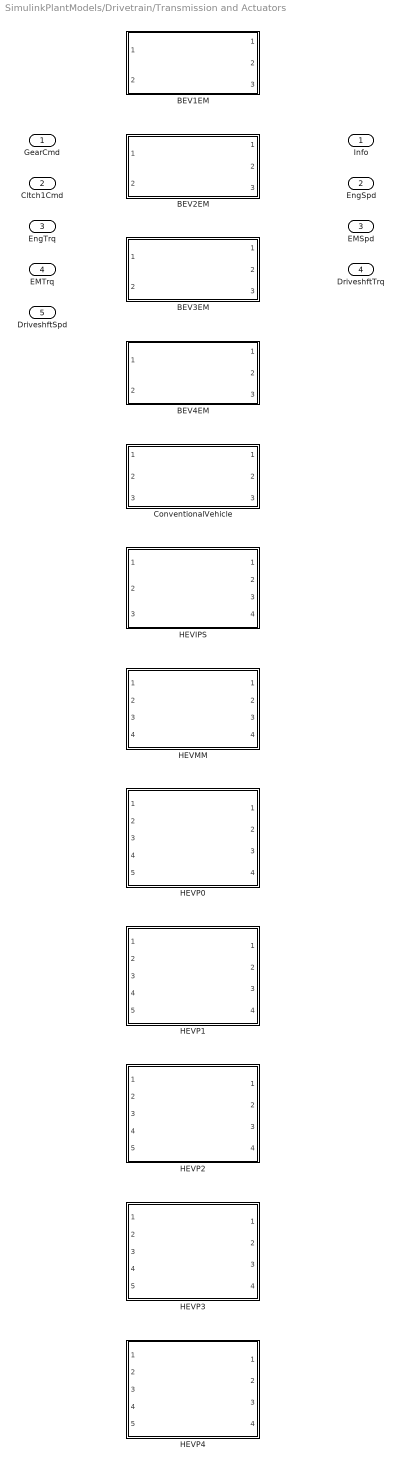
== system SimulinkPlantModels/Drivetrain/Transmission and Actuators ==
  GearCmd : Inport
  Cltch1Cmd : Inport  Port=2
  EngTrq : Inport  Port=3
  EMTrq : Inport  Port=4
  DriveshftSpd : Inport  Port=5
  BEV1EM : Subsystem  VariantControl=BEV1EM  ReferencedSubsystem=BEV1EM
  BEV2EM : Subsystem  VariantControl=BEV2EM  ReferencedSubsystem=BEV2EM
  BEV3EM : Subsystem  VariantControl=BEV3EM  ReferencedSubsystem=BEV3EM
  BEV4EM : Subsystem  VariantControl=BEV4EM  ReferencedSubsystem=BEV4EM
  ConventionalVehicle : Subsystem  VariantControl=ConventionalVehicle  ReferencedSubsystem=ConventionalVehicle
  HEVIPS : Subsystem  VariantControl=HEVIPS  ReferencedSubsystem=HEVIPS
  HEVMM : Subsystem  VariantControl=HEVMM  ReferencedSubsystem=HEVMM
  HEVP0 : Subsystem  VariantControl=HEVP0  ReferencedSubsystem=HEVP0
  HEVP1 : Subsystem  VariantControl=HEVP1  ReferencedSubsystem=HEVP1
  HEVP2 : Subsystem  VariantControl=HEVP2  ReferencedSubsystem=HEVP2
  HEVP3 : Subsystem  VariantControl=HEVP3  ReferencedSubsystem=HEVP3
  HEVP4 : Subsystem  VariantControl=HEVP4  ReferencedSubsystem=HEVP4
  Info : Outport  VectorParamsAs1DForOutWhenUnconnected=off
  EngSpd : Outport  Port=2  VectorParamsAs1DForOutWhenUnconnected=off
  EMSpd : Outport  Port=3  VectorParamsAs1DForOutWhenUnconnected=off  BusOutputAsStruct=on
  DriveshftTrq : Outport  Port=4  VectorParamsAs1DForOutWhenUnconnected=off

== system SimulinkPlantModels/Pedal, Cluster, Cabin/Brake Pedal ==
  DecelCmd : Inport
  Dead Zone1 : DeadZone  LowerValue=0  UpperValue=.01  ZeroCross=off
  DecelFdbk : Outport
  wires:
  Dead Zone1/1 -> DecelFdbk/1
  DecelCmd/1 -> Dead Zone1/1

== system SimulinkPlantModels/Sensors/Sensors ==
  VehFdbk : Inport
  IMUSensor : Subsystem  VariantControl=IMUSensor  ReferencedSubsystem=IMUSensor
  NoIMUSensor : Subsystem  VariantControl=NoIMUSensor  ReferencedSubsystem=NoIMUSensor
  IMU : Outport

== system SimulinkPlantModels/Thermal/Electrical Cooling ==
  No Thermal Effect : Subsystem  VariantControl=No Thermal Effect
  Thermal : Outport

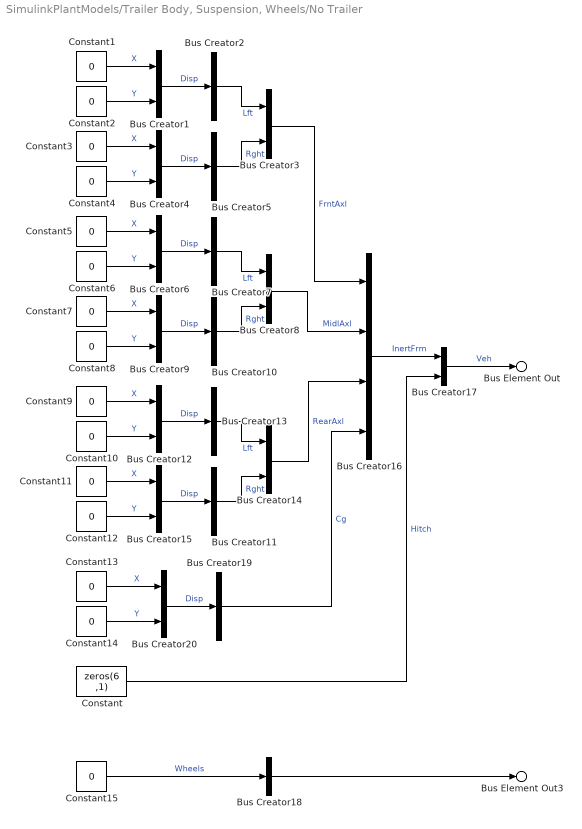
== system SimulinkPlantModels/Trailer Body, Suspension, Wheels/No Trailer ==
  Bus Creator{1,3..4,6,8..9,12,14..15,17,20} (11 alike) : BusCreator  Inputs=2
  Bus Creator{2,5,7,10..11,13,18..19} (8 alike) : BusCreator  Inputs=1
  Bus Creator16 : BusCreator  Inputs=4
  Constant : Constant  Value=zeros(6 ,1)  SampleTime=-1
  Constant{1..15} (15 alike) : Constant  Value=0  SampleTime=-1
  Bus Element Out3 : Outport  PortName=Wheels
  Bus Element Out : Outport  Port=2  PortName=Veh
  wires:
  Constant1/1 -> Bus Creator1/1  "X"
  Bus Creator18/1 -> Bus Element Out3/1
  Constant2/1 -> Bus Creator1/2  "Y"
  Bus Creator1/1 -> Bus Creator2/1  "Disp"
  Bus Creator4/1 -> Bus Creator5/1  "Disp"
  Constant4/1 -> Bus Creator4/2  "Y"
  Constant3/1 -> Bus Creator4/1  "X"
  Bus Creator5/1 -> Bus Creator3/2  "Rght"
  Bus Creator2/1 -> Bus Creator3/1  "Lft"
  Bus Creator7/1 -> Bus Creator8/1  "Lft"
  Bus Creator10/1 -> Bus Creator8/2  "Rght"
  Constant7/1 -> Bus Creator9/1  "X"
  Constant8/1 -> Bus Creator9/2  "Y"
  Bus Creator9/1 -> Bus Creator10/1  "Disp"
  Bus Creator6/1 -> Bus Creator7/1  "Disp"
  Constant6/1 -> Bus Creator6/2  "Y"
  Constant5/1 -> Bus Creator6/1  "X"
  Constant9/1 -> Bus Creator12/1  "X"
  Constant10/1 -> Bus Creator12/2  "Y"
  Bus Creator12/1 -> Bus Creator13/1  "Disp"
  Bus Creator15/1 -> Bus Creator11/1  "Disp"
  Constant12/1 -> Bus Creator15/2  "Y"
  Constant11/1 -> Bus Creator15/1  "X"
  Bus Creator11/1 -> Bus Creator14/2  "Rght"
  Bus Creator13/1 -> Bus Creator14/1  "Lft"
  Bus Creator8/1 -> Bus Creator16/2  "MidlAxl"
  Bus Creator14/1 -> Bus Creator16/3  "RearAxl"
  Bus Creator3/1 -> Bus Creator16/1  "FrntAxl"
  Bus Creator16/1 -> Bus Creator17/1  "InertFrm"
  Bus Creator17/1 -> Bus Element Out/1  "Veh"
  Constant15/1 -> Bus Creator18/1  "Wheels"
  Bus Creator19/1 -> Bus Creator16/4  "Cg"
  Constant13/1 -> Bus Creator20/1  "X"
  Constant14/1 -> Bus Creator20/2  "Y"
  Bus Creator20/1 -> Bus Creator19/1  "Disp"
  Constant/1 -> Bus Creator17/2  "Hitch"

== system SimulinkPlantModels/Body, Suspension, Wheels/Powertrain Bypass/External Signal Source ==
  note: User can insert any time based
      | wheel torque signal source here,
      | including 'From File' or 'From
      | Workspace' sources.
      |
      | Positive torque moves vehicle
      | forward.
      | Negative torque brakes forward
      | moving vehicle or moves vehicle
      | in reverse.
  note: Disables Pressure
      | Input for Brakes
  Constant{2..5} (4 alike) : Constant  Value=0  SampleTime=-1
  FL : Step  After=100  SampleTime=0
  FR : Step  After=100  SampleTime=0
  RL : Constant  Value=0  SampleTime=-1
  RR : Constant  Value=0  SampleTime=-1
  Vector Concatenate : Concatenate  NumInputs=4
  Vector Concatenate1 : Concatenate  NumInputs=4
  BrkPrsCmdOut : Outport
  AxlTrqOut : Outport  Port=2
  wires:
  FL/1 -> Vector Concatenate/1
  FR/1 -> Vector Concatenate/2
  RL/1 -> Vector Concatenate/3
  RR/1 -> Vector Concatenate/4
  Vector Concatenate/1 -> AxlTrqOut/1
  Constant2/1 -> Vector Concatenate1/1
  Constant3/1 -> Vector Concatenate1/2
  Constant4/1 -> Vector Concatenate1/3
  Vector Concatenate1/1 -> BrkPrsCmdOut/1
  Constant5/1 -> Vector Concatenate1/4

== system SimulinkPlantModels/Body, Suspension, Wheels/Powertrain Bypass/Pass Through ==
  BrkPrsCmdIn : Inport
  AlxTrqIn : Inport  Port=2
  BrkPrsCmdOut : Outport
  AxlTrqOut : Outport  Port=2
  wires:
  AlxTrqIn/1 -> AxlTrqOut/1
  BrkPrsCmdIn/1 -> BrkPrsCmdOut/1

== system SimulinkPlantModels/Drivetrain/Drivetrain Layout/Axle Interconnect ==
  TrqSplitRatio : Inport
  SpdLock : Inport  Port=2
  FrntDiffrntlSpd : Inport  Port=3
  DriveshftTrq : Inport  Port=4
  RearDiffrntlSpd : Inport  Port=5
  NoInterconnect : Subsystem  VariantControl=NoInterconnect  ReferencedSubsystem=NoInterconnect
  TransferCase : Subsystem  VariantControl=TransferCase  ReferencedSubsystem=TransferCase
  DriveshftSpd : Outport
  FrntDiffrntlTrq : Outport  Port=2
  RearDiffrntlTrq : Outport  Port=3

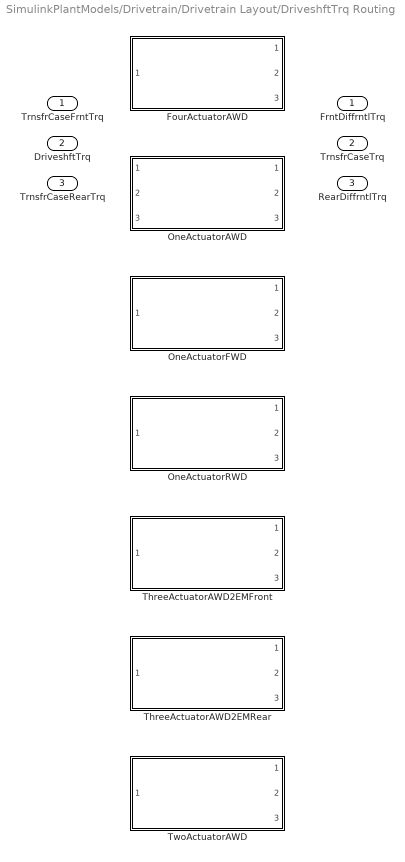
== system SimulinkPlantModels/Drivetrain/Drivetrain Layout/DriveshftTrq Routing ==
  TrnsfrCaseFrntTrq : Inport
  DriveshftTrq : Inport  Port=2
  "TrnsfrCaseRearTrq " : Inport  Port=3
  FourActuatorAWD : Subsystem  VariantControl=FourActuatorAWD  ReferencedSubsystem=FourActuatorAWD
  OneActuatorAWD : Subsystem  VariantControl=OneActuatorAWD  ReferencedSubsystem=OneActuatorAWD
  OneActuatorFWD : Subsystem  VariantControl=OneActuatorFWD  ReferencedSubsystem=OneActuatorFWD
  OneActuatorRWD : Subsystem  VariantControl=OneActuatorRWD  ReferencedSubsystem=OneActuatorRWD
  ThreeActuatorAWD2EMFront : Subsystem  VariantControl=ThreeActuatorAWD2EMFront  ReferencedSubsystem=ThreeActuatorAWD2EMFront
  ThreeActuatorAWD2EMRear : Subsystem  VariantControl=ThreeActuatorAWD2EMRear  ReferencedSubsystem=ThreeActuatorAWD2EMRear
  TwoActuatorAWD : Subsystem  VariantControl=TwoActuatorAWD  ReferencedSubsystem=TwoActuatorAWD
  FrntDiffrntlTrq : Outport
  TrnsfrCaseTrq : Outport  Port=2
  RearDiffrntlTrq : Outport  Port=3

== system SimulinkPlantModels/Drivetrain/Drivetrain Layout/Drivetrain Wheel Speed Route ==
  note: 1) Add Subsystem or Model blocks as valid variant choices.
      | 2) You cannot connect blocks at this level. At simulation, connectivity is automatically
      | determined, based on the active variant and port name matching.
  Omega : Inport
  Bus : Subsystem  VariantControl=Bus
  Vector : Subsystem  VariantControl=Vector
  Vector three-axle : Subsystem  VariantControl=Vector1
  Omega_LF : Outport
  Omega_RF : Outport  Port=2
  Omega_LR : Outport  Port=3
  Omega_RR : Outport  Port=4

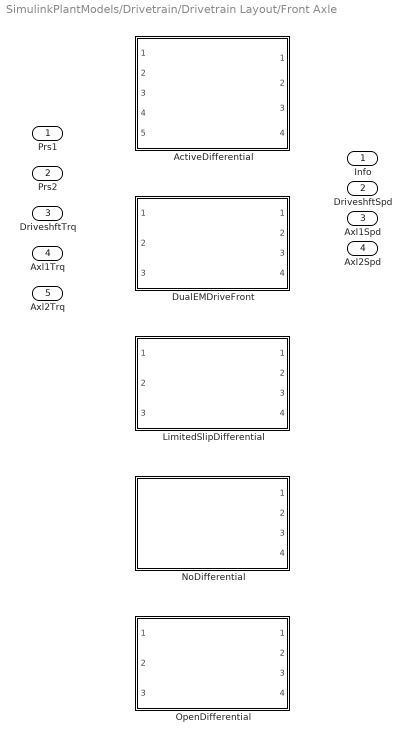
== system SimulinkPlantModels/Drivetrain/Drivetrain Layout/Front Axle ==
  Prs1 : Inport
  Prs2 : Inport  Port=2
  DriveshftTrq : Inport  Port=3
  Axl1Trq : Inport  Port=4
  Axl2Trq : Inport  Port=5
  ActiveDifferential : Subsystem  VariantControl=ActiveDifferential  ReferencedSubsystem=ActiveDifferential
  DualEMDriveFront : Subsystem  VariantControl=DualEMDriveFront  ReferencedSubsystem=DualEMDriveFront
  LimitedSlipDifferential : Subsystem  VariantControl=LimitedSlipDifferential  ReferencedSubsystem=LimitedSlipDifferential
  NoDifferential : Subsystem  VariantControl=NoDifferential  ReferencedSubsystem=NoDifferential
  OpenDifferential : Subsystem  VariantControl=OpenDifferential  ReferencedSubsystem=OpenDifferential
  Info : Outport
  DriveshftSpd : Outport  Port=2
  Axl1Spd : Outport  Port=3
  Axl2Spd : Outport  Port=4

== system SimulinkPlantModels/Drivetrain/Drivetrain Layout/Front Axle Compliances ==
  RSpdL : Inport
  RSpdR : Inport  Port=2
  OmegaL : Inport  Port=3
  OmegaR : Inport  Port=4
  AxleCompliances : Subsystem  VariantControl=AxleCompliances  ReferencedSubsystem=AxleCompliances
  NoAxleCompliances : Subsystem  VariantControl=NoAxleCompliances  ReferencedSubsystem=NoAxleCompliances
  RTrqL : Outport
  RTrqR : Outport  Port=2
  CTrqL : Outport  Port=3
  CTrqR : Outport  Port=4

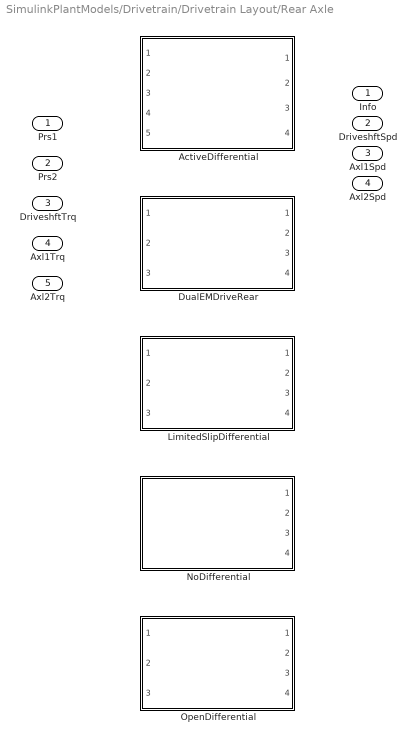
== system SimulinkPlantModels/Drivetrain/Drivetrain Layout/Rear Axle ==
  Prs1 : Inport
  Prs2 : Inport  Port=2
  DriveshftTrq : Inport  Port=3
  Axl1Trq : Inport  Port=4
  Axl2Trq : Inport  Port=5
  ActiveDifferential : Subsystem  VariantControl=ActiveDifferential  ReferencedSubsystem=ActiveDifferential
  DualEMDriveRear : Subsystem  VariantControl=DualEMDriveRear  ReferencedSubsystem=DualEMDriveRear
  LimitedSlipDifferential : Subsystem  VariantControl=LimitedSlipDifferential  ReferencedSubsystem=LimitedSlipDifferential
  NoDifferential : Subsystem  VariantControl=NoDifferential  ReferencedSubsystem=NoDifferential
  OpenDifferential : Subsystem  VariantControl=OpenDifferential  ReferencedSubsystem=OpenDifferential
  Info : Outport
  DriveshftSpd : Outport  Port=2
  Axl1Spd : Outport  Port=3
  Axl2Spd : Outport  Port=4

== system SimulinkPlantModels/Drivetrain/Drivetrain Layout/Rear Axle Compliances ==
  RSpdL : Inport
  RSpdR : Inport  Port=2
  OmegaL : Inport  Port=3
  OmegaR : Inport  Port=4
  AxleCompliances : Subsystem  VariantControl=AxleCompliances  ReferencedSubsystem=AxleCompliances
  NoAxleCompliances : Subsystem  VariantControl=NoAxleCompliances  ReferencedSubsystem=NoAxleCompliances
  CTrqL : Outport
  CTrqR : Outport  Port=2
  RTrqL : Outport  Port=3
  RTrqR : Outport  Port=4

== system SimulinkPlantModels/Drivetrain/Drivetrain Layout/Variant Subsystem ==
  note: 1) Add Subsystem or Model blocks as valid variant choices.
      | 2) You cannot connect blocks at this level. At simulation, connectivity is automatically
      | determined, based on the active variant and port name matching.
  FL : Inport
  FR : Inport  Port=2
  RL : Inport  Port=3
  RR : Inport  Port=4
  Three-axle output : Subsystem  VariantControl=ThreeAxleOutput
  Two-axle output : Subsystem  VariantControl=TwoAxleOutput
  AxlTrq : Outport

== system SimulinkPlantModels/Thermal/Electrical Cooling/No Thermal Effect ==
  Constant : Constant  Value=0  SampleTime=-1
  Constant1 : Constant  Value=0  SampleTime=-1
  Out Bus Element : Outport  PortName=Thermal  Element=EPumpPwr
  Out Bus Element1 : Outport  PortName=Thermal  Element=CoolTemp
  wires:
  Constant/1 -> Out Bus Element/1
  Constant1/1 -> Out Bus Element1/1

== system SimulinkPlantModels/Drivetrain/Drivetrain Layout/Drivetrain Wheel Speed Route/Bus ==
  Omega : Inport
  Bus Selector : BusSelector  OutputSignals=Omega_LF,Omega_RF,Omega_LR,Omega_RR
  Omega_LF : Outport
  Omega_RF : Outport  Port=2
  Omega_LR : Outport  Port=3
  Omega_RR : Outport  Port=4
  wires:
  Bus Selector/3 -> Omega_LR/1  "<Omega_LR>"
  Bus Selector/4 -> Omega_RR/1  "<Omega_RR>"
  Bus Selector/2 -> Omega_RF/1  "<Omega_RF>"
  Bus Selector/1 -> Omega_LF/1  "<Omega_LF>"
  Omega/1 -> Bus Selector/1

== system SimulinkPlantModels/Drivetrain/Drivetrain Layout/Drivetrain Wheel Speed Route/Vector ==
  Omega : Inport
  Demux : Demux
  Omega_LF : Outport
  Omega_RF : Outport  Port=2
  Omega_LR : Outport  Port=3
  Omega_RR : Outport  Port=4
  wires:
  Demux/2 -> Omega_RF/1
  Demux/1 -> Omega_LF/1
  Demux/3 -> Omega_LR/1
  Omega/1 -> Demux/1
  Demux/4 -> Omega_RR/1

== system SimulinkPlantModels/Drivetrain/Drivetrain Layout/Drivetrain Wheel Speed Route/Vector three-axle ==
  Omega : Inport
  Demux : Demux  Outputs=6
  Terminator : Terminator
  Terminator1 : Terminator
  Omega_LF : Outport
  Omega_RF : Outport  Port=2
  Omega_LR : Outport  Port=3
  Omega_RR : Outport  Port=4
  wires:
  Demux/2 -> Omega_RF/1
  Demux/1 -> Omega_LF/1
  Demux/5 -> Omega_LR/1
  Omega/1 -> Demux/1
  Demux/6 -> Omega_RR/1
  Demux/3 -> Terminator/1
  Demux/4 -> Terminator1/1

== system SimulinkPlantModels/Drivetrain/Drivetrain Layout/Variant Subsystem/Three-axle output ==
  FL : Inport
  FR : Inport  Port=2
  RL : Inport  Port=3
  RR : Inport  Port=4
  Bus Creator : BusCreator  Inputs=6
  Gain : Gain
  Gain1 : Gain
  AxlTrq : Outport
  wires:
  FL/1 -> Bus Creator/1
  FR/1 -> Bus Creator/2
  RR/1 -> Gain1/1, Bus Creator/6
  Bus Creator/1 -> AxlTrq/1  "AxlTrq"
  Gain/1 -> Bus Creator/3  "ML"
  RL/1 -> Gain/1, Bus Creator/5
  Gain1/1 -> Bus Creator/4  "MR"

== system SimulinkPlantModels/Drivetrain/Drivetrain Layout/Variant Subsystem/Two-axle output ==
  FL : Inport
  FR : Inport  Port=2
  RL : Inport  Port=3
  RR : Inport  Port=4
  Bus Creator : BusCreator  Inputs=4
  AxlTrq : Outport
  wires:
  FL/1 -> Bus Creator/1  "FL"
  FR/1 -> Bus Creator/2  "FR"
  RR/1 -> Bus Creator/4  "RR"
  Bus Creator/1 -> AxlTrq/1  "AxlTrq"
  RL/1 -> Bus Creator/3  "RL"
